simulink model "ssc_Probes_test_all_16a"  (R2019b)
settings: Solver=ode23t  StartTime=0.0  StopTime=10.0  RelTol=1e-3  EnableMultiTasking=on
undefined symbols (not defined in the file): damping_coeff
libraries: fl_lib x88, nesl_utility x71, Pneumatic_lib x16, fl_ps_legacy_lib x1
(part 3 of 4)

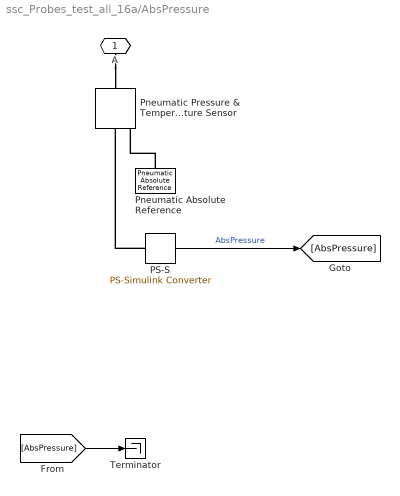
== system ssc_Probes_test_all_16a/AbsPressure ==
  PS-S : nesl_utility/PS-Simulink Converter  PhysicalDomain=network_engine_domain  SubClassName=ps_output  LeftPortType=input  RightPortType=output  PseudoPeriodic=off  Frequencies=[]  Unit=Pa  AffineConversion=off
  Pneumatic Absolute Reference : Pneumatic_lib/Pneumatic Elements/Pneumatic Absolute Reference
      settings: InternalSimscapePortConfiguration="{\"Bottom\":[],\"Left\":[{\"id\":\"A\",\"label\":\"\",\"type\":\"foundation.pneumatic.pneumatic\"}],\"Right\":[],\"Top\":[]}"
  Pneumatic Pressure & Temperature Sensor : Pneumatic_lib/Pneumatic Sensors/Pneumatic Pressure & Temperature Sensor
      settings: InternalSimscapePortConfiguration="{\"Bottom\":[],\"Left\":[{\"id\":\"A\",\"label\":\"A\",\"type\":\"foundation.pneumatic.pneumatic\"}],\"Right\":[{\"id\":\"B\",\"label\":\"B\",\"type\":\"foundation.pneumatic.pneumatic\"},{\"id\":\"P_ps\",\"label\":\"P\",\"type\":\"output\"},{\"id\":\"T_ps\",\"label\":\"T\",\"type\":\"output\"}],\"Top\":[]}"
  Terminator : Terminator
  A : PMIOPort  Side=Left
  wires:
  [AbsPressure] -> Terminator/1
  PS-S/1 -> [AbsPressure]  "AbsPressure"
  connections:
  PS-S/LConn1 -- Pneumatic Pressure & Temperature Sensor/RConn2
  Pneumatic Absolute Reference/LConn1 -- Pneumatic Pressure & Temperature Sensor/RConn1
  A/RConn1 -- Pneumatic Pressure & Temperature Sensor/LConn1

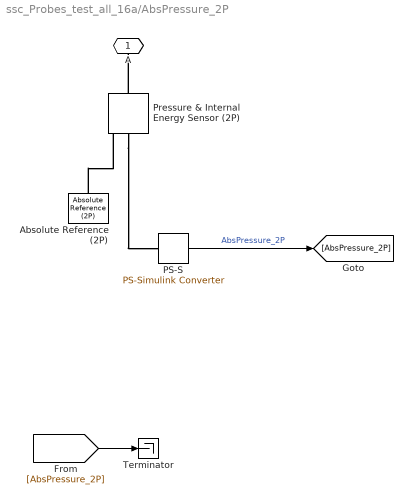
== system ssc_Probes_test_all_16a/AbsPressure_2P ==
  Absolute Reference (2P) : fl_lib/Two-Phase Fluid/Elements/Absolute Reference (2P)
      settings: SourceProductName=Simscape  SourceProductBaseCode=SS
  PS-S : nesl_utility/PS-Simulink Converter  PhysicalDomain=network_engine_domain  SubClassName=ps_output  LeftPortType=input  RightPortType=output  PseudoPeriodic=off  Frequencies=[]  Unit=Pa  AffineConversion=off
  Pressure & Internal Energy Sensor (2P) : fl_lib/Two-Phase Fluid/Sensors/Pressure & Internal Energy Sensor (2P)
      settings: SourceProductName=Simscape  SourceProductBaseCode=SS  InternalSimscapePortConfiguration="{\"Bottom\":[],\"Left\":[{\"id\":\"A\",\"label\":\"A\",\"type\":\"foundation.two_phase_fluid.two_phase_fluid\"}],\"Right\":[{\"id\":\"B\",\"label\":\"B\",\"type\":\"foundation.two_phase_fluid.two_phase_fluid\"},{\"id\":\"P\",\"label\":\"P\",\"type\":\"output\"},{\"id\":\"U\",\"label\":\"U\",\"type\":\"output\"}],\"Top\":[]}"
  Terminator : Terminator
  A : PMIOPort  Side=Left
  wires:
  [AbsPressure_2P] -> Terminator/1
  PS-S/1 -> [AbsPressure_2P]  "AbsPressure_2P"
  connections:
  Absolute Reference (2P)/LConn1 -- Pressure & Internal Energy Sensor (2P)/RConn1
  Pressure & Internal Energy Sensor (2P)/RConn2 -- PS-S/LConn1
  Pressure & Internal Energy Sensor (2P)/LConn1 -- A/RConn1

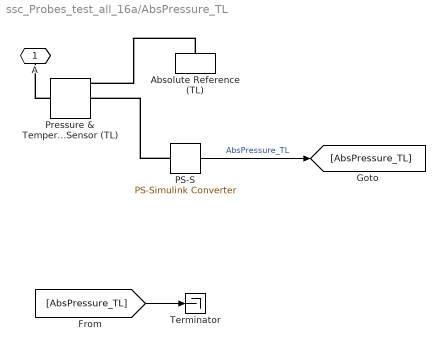
== system ssc_Probes_test_all_16a/AbsPressure_TL ==
  Absolute Reference (TL) : fl_lib/Thermal Liquid/Elements/Absolute Reference (TL)
      settings: SourceProductName=Simscape  SourceProductBaseCode=SS
  PS-S : nesl_utility/PS-Simulink Converter  PhysicalDomain=network_engine_domain  SubClassName=ps_output  LeftPortType=input  RightPortType=output  PseudoPeriodic=off  Frequencies=[]  Unit=Pa  AffineConversion=off
  Pressure & Temperature Sensor (TL) : fl_lib/Thermal Liquid/Sensors/Pressure & Temperature Sensor (TL)
      settings: SourceProductName=Simscape  SourceProductBaseCode=SS  InternalSimscapePortConfiguration="{\"Bottom\":[],\"Left\":[{\"id\":\"A\",\"label\":\"A\",\"type\":\"foundation.thermal_liquid.thermal_liquid\"}],\"Right\":[{\"id\":\"B\",\"label\":\"B\",\"type\":\"foundation.thermal_liquid.thermal_liquid\"},{\"id\":\"P\",\"label\":\"P\",\"type\":\"output\"},{\"id\":\"T\",\"label\":\"T\",\"type\":\"output\"}],\"Top\":[]}"
  Terminator : Terminator
  A : PMIOPort  Side=Left
  wires:
  [AbsPressure_TL] -> Terminator/1
  PS-S/1 -> [AbsPressure_TL]  "AbsPressure_TL"
  connections:
  PS-S/LConn1 -- Pressure & Temperature Sensor (TL)/RConn2
  Pressure & Temperature Sensor (TL)/LConn1 -- A/RConn1
  Absolute Reference (TL)/LConn1 -- Pressure & Temperature Sensor (TL)/RConn1

== system ssc_Probes_test_all_16a/AbsTemp_2P ==
  PS-S : nesl_utility/PS-Simulink Converter  PhysicalDomain=network_engine_domain  SubClassName=ps_output  LeftPortType=input  RightPortType=output  PseudoPeriodic=off  Frequencies=[]  Unit=K  AffineConversion=off
  Terminator : Terminator
  Thermodynamic Properties Sensor (2P) : fl_lib/Two-Phase Fluid/Sensors/Thermodynamic Properties Sensor (2P)
      settings: SourceProductName=Simscape  SourceProductBaseCode=SS  InternalSimscapePortConfiguration="{\"Bottom\":[],\"Left\":[{\"id\":\"A\",\"label\":\"A\",\"type\":\"foundation.two_phase_fluid.two_phase_fluid\"}],\"Right\":[{\"id\":\"T\",\"label\":\"T\",\"type\":\"output\"},{\"id\":\"H\",\"label\":\"h\",\"type\":\"output\"},{\"id\":\"V\",\"label\":\"v\",\"type\":\"output\"},{\"id\":\"S\",\"label\":\"s\",\"type\":\"output\"}],\"Top\":[]}"
  A : PMIOPort  Side=Left
  wires:
  PS-S/1 -> [AbsTemp_2P]  "AbsTemp_2P"
  [AbsTemp_2P] -> Terminator/1
  connections:
  A/RConn1 -- Thermodynamic Properties Sensor (2P)/LConn1
  Thermodynamic Properties Sensor (2P)/RConn1 -- PS-S/LConn1

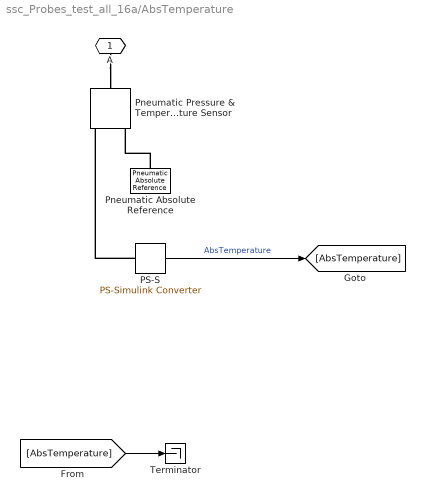
== system ssc_Probes_test_all_16a/AbsTemperature ==
  PS-S : nesl_utility/PS-Simulink Converter  PhysicalDomain=network_engine_domain  SubClassName=ps_output  LeftPortType=input  RightPortType=output  PseudoPeriodic=off  Frequencies=[]  Unit=K  AffineConversion=off
  Pneumatic Absolute Reference : Pneumatic_lib/Pneumatic Elements/Pneumatic Absolute Reference
      settings: InternalSimscapePortConfiguration="{\"Bottom\":[],\"Left\":[{\"id\":\"A\",\"label\":\"\",\"type\":\"foundation.pneumatic.pneumatic\"}],\"Right\":[],\"Top\":[]}"
  Pneumatic Pressure & Temperature Sensor : Pneumatic_lib/Pneumatic Sensors/Pneumatic Pressure & Temperature Sensor
      settings: InternalSimscapePortConfiguration="{\"Bottom\":[],\"Left\":[{\"id\":\"A\",\"label\":\"A\",\"type\":\"foundation.pneumatic.pneumatic\"}],\"Right\":[{\"id\":\"B\",\"label\":\"B\",\"type\":\"foundation.pneumatic.pneumatic\"},{\"id\":\"P_ps\",\"label\":\"P\",\"type\":\"output\"},{\"id\":\"T_ps\",\"label\":\"T\",\"type\":\"output\"}],\"Top\":[]}"
  Terminator : Terminator
  A : PMIOPort  Side=Left
  wires:
  [AbsTemperature] -> Terminator/1
  PS-S/1 -> [AbsTemperature]  "AbsTemperature"
  connections:
  A/RConn1 -- Pneumatic Pressure & Temperature Sensor/LConn1
  Pneumatic Absolute Reference/LConn1 -- Pneumatic Pressure & Temperature Sensor/RConn1
  PS-S/LConn1 -- Pneumatic Pressure & Temperature Sensor/RConn3

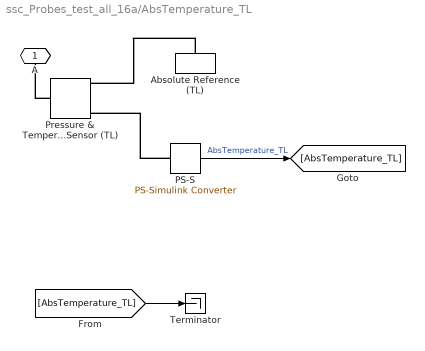
== system ssc_Probes_test_all_16a/AbsTemperature_TL ==
  Absolute Reference (TL) : fl_lib/Thermal Liquid/Elements/Absolute Reference (TL)
      settings: SourceProductName=Simscape  SourceProductBaseCode=SS
  PS-S : nesl_utility/PS-Simulink Converter  PhysicalDomain=network_engine_domain  SubClassName=ps_output  LeftPortType=input  RightPortType=output  PseudoPeriodic=off  Frequencies=[]  Unit=K  AffineConversion=off
  Pressure & Temperature Sensor (TL) : fl_lib/Thermal Liquid/Sensors/Pressure & Temperature Sensor (TL)
      settings: SourceProductName=Simscape  SourceProductBaseCode=SS  InternalSimscapePortConfiguration="{\"Bottom\":[],\"Left\":[{\"id\":\"A\",\"label\":\"A\",\"type\":\"foundation.thermal_liquid.thermal_liquid\"}],\"Right\":[{\"id\":\"B\",\"label\":\"B\",\"type\":\"foundation.thermal_liquid.thermal_liquid\"},{\"id\":\"P\",\"label\":\"P\",\"type\":\"output\"},{\"id\":\"T\",\"label\":\"T\",\"type\":\"output\"}],\"Top\":[]}"
  Terminator : Terminator
  A : PMIOPort  Side=Left
  wires:
  PS-S/1 -> [AbsTemperature_TL]  "AbsTemperature_TL"
  [AbsTemperature_TL] -> Terminator/1
  connections:
  Absolute Reference (TL)/LConn1 -- Pressure & Temperature Sensor (TL)/RConn1
  Pressure & Temperature Sensor (TL)/LConn1 -- A/RConn1
  PS-S/LConn1 -- Pressure & Temperature Sensor (TL)/RConn3

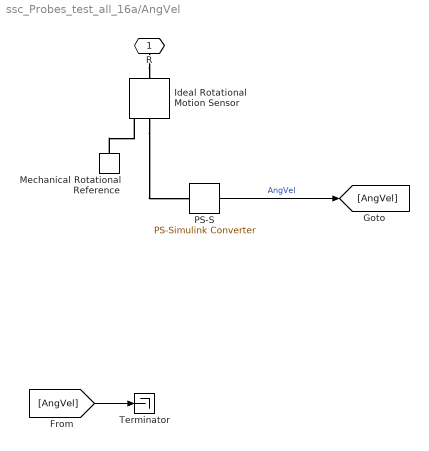
== system ssc_Probes_test_all_16a/AngVel ==
  Ideal Rotational Motion Sensor : fl_lib/Mechanical/Mechanical Sensors/Ideal Rotational Motion Sensor  offset=0 rad
  Mechanical Rotational Reference : fl_lib/Mechanical/Rotational Elements/Mechanical Rotational Reference
  PS-S : nesl_utility/PS-Simulink Converter  PhysicalDomain=network_engine_domain  SubClassName=ps_output  LeftPortType=input  RightPortType=output  PseudoPeriodic=off  Frequencies=[]  Unit=rad/s  AffineConversion=off
  Terminator : Terminator
  R : PMIOPort  Side=Left
  wires:
  [AngVel] -> Terminator/1
  PS-S/1 -> [AngVel]  "AngVel"
  connections:
  R/RConn1 -- Ideal Rotational Motion Sensor/LConn1
  Mechanical Rotational Reference/LConn1 -- Ideal Rotational Motion Sensor/RConn1
  Ideal Rotational Motion Sensor/RConn2 -- PS-S/LConn1

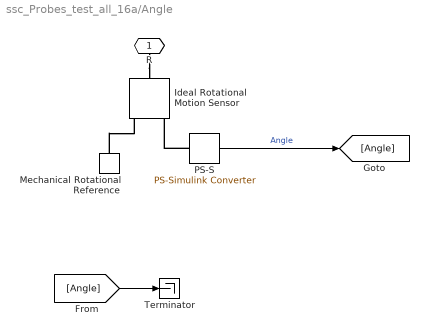
== system ssc_Probes_test_all_16a/Angle ==
  Ideal Rotational Motion Sensor : fl_lib/Mechanical/Mechanical Sensors/Ideal Rotational Motion Sensor  offset=0 rad
  Mechanical Rotational Reference : fl_lib/Mechanical/Rotational Elements/Mechanical Rotational Reference
  PS-S : nesl_utility/PS-Simulink Converter  PhysicalDomain=network_engine_domain  SubClassName=ps_output  LeftPortType=input  RightPortType=output  PseudoPeriodic=off  Frequencies=[]  Unit=rad  AffineConversion=off
  Terminator : Terminator
  R : PMIOPort  Side=Left
  wires:
  [Angle] -> Terminator/1
  PS-S/1 -> [Angle]  "Angle"
  connections:
  PS-S/LConn1 -- Ideal Rotational Motion Sensor/RConn3
  Mechanical Rotational Reference/LConn1 -- Ideal Rotational Motion Sensor/RConn1
  R/RConn1 -- Ideal Rotational Motion Sensor/LConn1

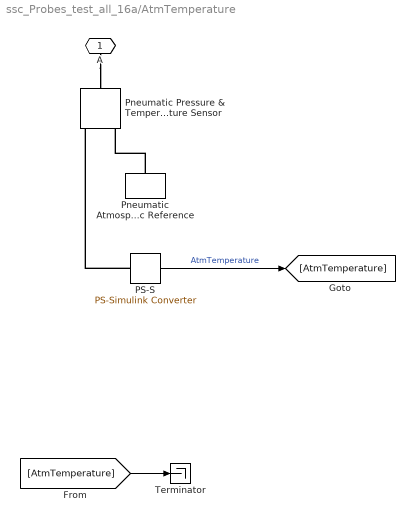
== system ssc_Probes_test_all_16a/AtmTemperature ==
  PS-S : nesl_utility/PS-Simulink Converter  PhysicalDomain=network_engine_domain  SubClassName=ps_output  LeftPortType=input  RightPortType=output  PseudoPeriodic=off  Frequencies=[]  Unit=K  AffineConversion=off
  Pneumatic Atmospheric Reference : Pneumatic_lib/Pneumatic Elements/Pneumatic Atmospheric Reference
      settings: InternalSimscapePortConfiguration="{\"Bottom\":[],\"Left\":[{\"id\":\"A\",\"label\":\"\",\"type\":\"foundation.pneumatic.pneumatic\"}],\"Right\":[],\"Top\":[]}"
  Pneumatic Pressure & Temperature Sensor : Pneumatic_lib/Pneumatic Sensors/Pneumatic Pressure & Temperature Sensor
      settings: InternalSimscapePortConfiguration="{\"Bottom\":[],\"Left\":[{\"id\":\"A\",\"label\":\"A\",\"type\":\"foundation.pneumatic.pneumatic\"}],\"Right\":[{\"id\":\"B\",\"label\":\"B\",\"type\":\"foundation.pneumatic.pneumatic\"},{\"id\":\"P_ps\",\"label\":\"P\",\"type\":\"output\"},{\"id\":\"T_ps\",\"label\":\"T\",\"type\":\"output\"}],\"Top\":[]}"
  Terminator : Terminator
  A : PMIOPort  Side=Left
  wires:
  [AtmTemperature] -> Terminator/1
  PS-S/1 -> [AtmTemperature]  "AtmTemperature"
  connections:
  PS-S/LConn1 -- Pneumatic Pressure & Temperature Sensor/RConn3
  Pneumatic Atmospheric Reference/LConn1 -- Pneumatic Pressure & Temperature Sensor/RConn1
  A/RConn1 -- Pneumatic Pressure & Temperature Sensor/LConn1

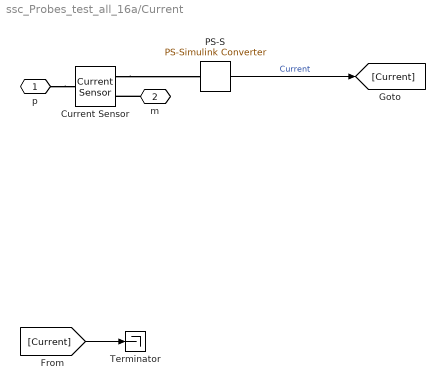
== system ssc_Probes_test_all_16a/Current ==
  Current Sensor : fl_lib/Electrical/Electrical Sensors/Current Sensor
  PS-S : nesl_utility/PS-Simulink Converter  PhysicalDomain=network_engine_domain  SubClassName=ps_output  LeftPortType=input  RightPortType=output  PseudoPeriodic=off  Frequencies=[]  Unit=A  AffineConversion=off
  Terminator : Terminator
  p : PMIOPort  Side=Left
  m : PMIOPort  Port=2  Side=Right
  wires:
  [Current] -> Terminator/1
  PS-S/1 -> [Current]  "Current"
  connections:
  Current Sensor/RConn1 -- PS-S/LConn1
  p/RConn1 -- Current Sensor/LConn1
  m/RConn1 -- Current Sensor/RConn2

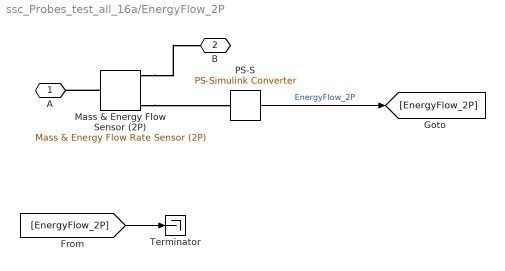
== system ssc_Probes_test_all_16a/EnergyFlow_2P ==
  Mass & Energy Flow Sensor (2P) : fl_lib/Two-Phase Fluid/Sensors/Mass & Energy Flow Rate Sensor (2P)
      settings: SourceProductName=Simscape  SourceProductBaseCode=SS  InternalSimscapePortConfiguration="{\"Bottom\":[],\"Left\":[{\"id\":\"A\",\"label\":\"A\",\"type\":\"foundation.two_phase_fluid.two_phase_fluid\"}],\"Right\":[{\"id\":\"B\",\"label\":\"B\",\"type\":\"foundation.two_phase_fluid.two_phase_fluid\"},{\"id\":\"M\",\"label\":\"M\",\"type\":\"output\"},{\"id\":\"PHI\",\"label\":\"Phi\",\"type\":\"output\"}],\"Top\":[]}"
  PS-S : nesl_utility/PS-Simulink Converter  PhysicalDomain=network_engine_domain  SubClassName=ps_output  LeftPortType=input  RightPortType=output  PseudoPeriodic=off  Frequencies=[]  Unit=kW  AffineConversion=off
  Terminator : Terminator
  A : PMIOPort  Side=Left
  B : PMIOPort  Port=2  Side=Right
  wires:
  [EnergyFlow_2P] -> Terminator/1
  PS-S/1 -> [EnergyFlow_2P]  "EnergyFlow_2P"
  connections:
  Mass & Energy Flow Sensor (2P)/RConn1 -- B/RConn1
  Mass & Energy Flow Sensor (2P)/RConn3 -- PS-S/LConn1
  Mass & Energy Flow Sensor (2P)/LConn1 -- A/RConn1

== system ssc_Probes_test_all_16a/Enthalpy_2P ==
  PS-S : nesl_utility/PS-Simulink Converter  PhysicalDomain=network_engine_domain  SubClassName=ps_output  LeftPortType=input  RightPortType=output  PseudoPeriodic=off  Frequencies=[]  Unit=kJ/kg  AffineConversion=off
  Terminator : Terminator
  Thermodynamic Properties Sensor (2P) : fl_lib/Two-Phase Fluid/Sensors/Thermodynamic Properties Sensor (2P)
      settings: SourceProductName=Simscape  SourceProductBaseCode=SS  InternalSimscapePortConfiguration="{\"Bottom\":[],\"Left\":[{\"id\":\"A\",\"label\":\"A\",\"type\":\"foundation.two_phase_fluid.two_phase_fluid\"}],\"Right\":[{\"id\":\"T\",\"label\":\"T\",\"type\":\"output\"},{\"id\":\"H\",\"label\":\"h\",\"type\":\"output\"},{\"id\":\"V\",\"label\":\"v\",\"type\":\"output\"},{\"id\":\"S\",\"label\":\"s\",\"type\":\"output\"}],\"Top\":[]}"
  A : PMIOPort  Side=Left
  wires:
  [Enthalpy_2P] -> Terminator/1
  PS-S/1 -> [Enthalpy_2P]  "Enthalpy_2P"
  connections:
  Thermodynamic Properties Sensor (2P)/RConn2 -- PS-S/LConn1
  A/RConn1 -- Thermodynamic Properties Sensor (2P)/LConn1

== system ssc_Probes_test_all_16a/Flow ==
  Ideal Hydraulic Flow Rate Sensor : fl_lib/Hydraulic/Hydraulic Sensors/Hydraulic Flow Rate Sensor
      settings: SourceProductName=Simscape
  PS-S : nesl_utility/PS-Simulink Converter  PhysicalDomain=network_engine_domain  SubClassName=ps_output  LeftPortType=input  RightPortType=output  PseudoPeriodic=off  Frequencies=[]  Unit=m^3/s  AffineConversion=off
  Terminator : Terminator
  A : PMIOPort  Side=Left
  B : PMIOPort  Port=2  Side=Right
  wires:
  [Flow] -> Terminator/1
  PS-S/1 -> [Flow]  "Flow"
  connections:
  A/RConn1 -- Ideal Hydraulic Flow Rate Sensor/LConn1
  Ideal Hydraulic Flow Rate Sensor/RConn1 -- PS-S/LConn1
  B/RConn1 -- Ideal Hydraulic Flow Rate Sensor/RConn2

== system ssc_Probes_test_all_16a/Flux ==
  Flux Sensor : fl_lib/Magnetic/Magnetic Sensors/Flux Sensor
      settings: SourceProductName=Simscape  SourceProductBaseCode=SS  InternalSimscapePortConfiguration="{\"Bottom\":[],\"Left\":[{\"id\":\"N\",\"label\":\"N\",\"type\":\"foundation.magnetic.magnetic\"}],\"Right\":[{\"id\":\"PHI\",\"label\":\"\",\"type\":\"output\"},{\"id\":\"S\",\"label\":\"S\",\"type\":\"foundation.magnetic.magnetic\"}],\"Top\":[]}"
  PS-S : nesl_utility/PS-Simulink Converter  PhysicalDomain=network_engine_domain  SubClassName=ps_output  LeftPortType=input  RightPortType=output  PseudoPeriodic=off  Frequencies=[]  Unit=Wb  AffineConversion=off
  Terminator : Terminator
  N : PMIOPort  Side=Left
  S : PMIOPort  Port=2  Side=Right
  wires:
  [Flux] -> Terminator/1
  PS-S/1 -> [Flux]  "Flux"
  connections:
  S/RConn1 -- Flux Sensor/RConn2
  Flux Sensor/RConn1 -- PS-S/LConn1
  N/RConn1 -- Flux Sensor/LConn1

== system ssc_Probes_test_all_16a/Force ==
  Ideal Force Sensor : fl_lib/Mechanical/Mechanical Sensors/Ideal Force Sensor
  PS-S : nesl_utility/PS-Simulink Converter  PhysicalDomain=network_engine_domain  SubClassName=ps_output  LeftPortType=input  RightPortType=output  PseudoPeriodic=off  Frequencies=[]  Unit=N  AffineConversion=off
  Terminator : Terminator
  R : PMIOPort  Side=Left
  C : PMIOPort  Port=2  Side=Right
  wires:
  [Force] -> Terminator/1
  PS-S/1 -> [Force]  "Force"
  connections:
  R/RConn1 -- Ideal Force Sensor/LConn1
  Ideal Force Sensor/RConn2 -- PS-S/LConn1
  C/RConn1 -- Ideal Force Sensor/RConn1

== system ssc_Probes_test_all_16a/GasHeatFlow ==
  PS-S : nesl_utility/PS-Simulink Converter  PhysicalDomain=network_engine_domain  SubClassName=ps_output  LeftPortType=input  RightPortType=output  PseudoPeriodic=off  Frequencies=[]  Unit=J/s  AffineConversion=off
  Pneumatic Mass & Heat Flow Sensor : Pneumatic_lib/Pneumatic Sensors/Pneumatic Mass & Heat Flow Sensor
      settings: InternalSimscapePortConfiguration="{\"Bottom\":[],\"Left\":[{\"id\":\"A\",\"label\":\"A\",\"type\":\"foundation.pneumatic.pneumatic\"}],\"Right\":[{\"id\":\"B\",\"label\":\"B\",\"type\":\"foundation.pneumatic.pneumatic\"},{\"id\":\"G_ps\",\"label\":\"G\",\"type\":\"output\"},{\"id\":\"Q_ps\",\"label\":\"Q\",\"type\":\"output\"}],\"Top\":[]}"
  Terminator : Terminator
  A : PMIOPort  Side=Left
  B : PMIOPort  Port=2  Side=Right
  wires:
  [GasHeatFlow] -> Terminator/1
  PS-S/1 -> [GasHeatFlow]  "GasHeatFlow"
  connections:
  A/RConn1 -- Pneumatic Mass & Heat Flow Sensor/LConn1
  B/RConn1 -- Pneumatic Mass & Heat Flow Sensor/RConn1
  PS-S/LConn1 -- Pneumatic Mass & Heat Flow Sensor/RConn3

== system ssc_Probes_test_all_16a/GaugePressure ==
  PS-S : nesl_utility/PS-Simulink Converter  PhysicalDomain=network_engine_domain  SubClassName=ps_output  LeftPortType=input  RightPortType=output  PseudoPeriodic=off  Frequencies=[]  Unit=Pa  AffineConversion=off
  Pneumatic Atmospheric Reference : Pneumatic_lib/Pneumatic Elements/Pneumatic Atmospheric Reference
      settings: InternalSimscapePortConfiguration="{\"Bottom\":[],\"Left\":[{\"id\":\"A\",\"label\":\"\",\"type\":\"foundation.pneumatic.pneumatic\"}],\"Right\":[],\"Top\":[]}"
  Pneumatic Pressure & Temperature Sensor : Pneumatic_lib/Pneumatic Sensors/Pneumatic Pressure & Temperature Sensor
      settings: InternalSimscapePortConfiguration="{\"Bottom\":[],\"Left\":[{\"id\":\"A\",\"label\":\"A\",\"type\":\"foundation.pneumatic.pneumatic\"}],\"Right\":[{\"id\":\"B\",\"label\":\"B\",\"type\":\"foundation.pneumatic.pneumatic\"},{\"id\":\"P_ps\",\"label\":\"P\",\"type\":\"output\"},{\"id\":\"T_ps\",\"label\":\"T\",\"type\":\"output\"}],\"Top\":[]}"
  Terminator : Terminator
  A : PMIOPort  Side=Left
  wires:
  [GaugePressure] -> Terminator/1
  PS-S/1 -> [GaugePressure]  "GaugePressure"
  connections:
  A/RConn1 -- Pneumatic Pressure & Temperature Sensor/LConn1
  Pneumatic Atmospheric Reference/LConn1 -- Pneumatic Pressure & Temperature Sensor/RConn1
  PS-S/LConn1 -- Pneumatic Pressure & Temperature Sensor/RConn2

== system ssc_Probes_test_all_16a/HeatFlow ==
  Ideal Heat Flow Sensor : fl_lib/Thermal/Thermal Sensors/Heat Flow Rate Sensor
      settings: SourceProductName=Simscape  SourceProductBaseCode=SS
  PS-S : nesl_utility/PS-Simulink Converter  PhysicalDomain=network_engine_domain  SubClassName=ps_output  LeftPortType=input  RightPortType=output  PseudoPeriodic=off  Frequencies=[]  Unit=J/s  AffineConversion=off
  Terminator : Terminator
  A : PMIOPort  Side=Left
  B : PMIOPort  Port=2  Side=Right
  wires:
  [HeatFlow] -> Terminator/1
  PS-S/1 -> [HeatFlow]  "HeatFlow"
  connections:
  B/RConn1 -- Ideal Heat Flow Sensor/RConn2
  Ideal Heat Flow Sensor/RConn1 -- PS-S/LConn1
  A/RConn1 -- Ideal Heat Flow Sensor/LConn1

== system ssc_Probes_test_all_16a/InternalEnergy_2P ==
  Absolute Reference (2P) : fl_lib/Two-Phase Fluid/Elements/Absolute Reference (2P)
      settings: SourceProductName=Simscape  SourceProductBaseCode=SS
  PS-S : nesl_utility/PS-Simulink Converter  PhysicalDomain=network_engine_domain  SubClassName=ps_output  LeftPortType=input  RightPortType=output  PseudoPeriodic=off  Frequencies=[]  Unit=kJ/kg  AffineConversion=off
  Pressure & Internal Energy Sensor (2P) : fl_lib/Two-Phase Fluid/Sensors/Pressure & Internal Energy Sensor (2P)
      settings: SourceProductName=Simscape  SourceProductBaseCode=SS  InternalSimscapePortConfiguration="{\"Bottom\":[],\"Left\":[{\"id\":\"A\",\"label\":\"A\",\"type\":\"foundation.two_phase_fluid.two_phase_fluid\"}],\"Right\":[{\"id\":\"B\",\"label\":\"B\",\"type\":\"foundation.two_phase_fluid.two_phase_fluid\"},{\"id\":\"P\",\"label\":\"P\",\"type\":\"output\"},{\"id\":\"U\",\"label\":\"U\",\"type\":\"output\"}],\"Top\":[]}"
  Terminator : Terminator
  A : PMIOPort  Side=Left
  wires:
  PS-S/1 -> [InternalEnergy_2P]  "InternalEnergy_2P"
  [InternalEnergy_2P] -> Terminator/1
  connections:
  Pressure & Internal Energy Sensor (2P)/LConn1 -- A/RConn1
  Pressure & Internal Energy Sensor (2P)/RConn3 -- PS-S/LConn1
  Absolute Reference (2P)/LConn1 -- Pressure & Internal Energy Sensor (2P)/RConn1

== system ssc_Probes_test_all_16a/MMF ==
  MMF Sensor : fl_lib/Magnetic/Magnetic Sensors/MMF Sensor
      settings: SourceProductName=Simscape  SourceProductBaseCode=SS  InternalSimscapePortConfiguration="{\"Bottom\":[],\"Left\":[{\"id\":\"N\",\"label\":\"N\",\"type\":\"foundation.magnetic.magnetic\"}],\"Right\":[{\"id\":\"MMF\",\"label\":\"\",\"type\":\"output\"},{\"id\":\"S\",\"label\":\"S\",\"type\":\"foundation.magnetic.magnetic\"}],\"Top\":[]}"
  Magnetic Reference : fl_lib/Magnetic/Magnetic Elements/Magnetic Reference
      settings: SourceProductName=Simscape  SourceProductBaseCode=SS  InternalSimscapePortConfiguration="{\"Bottom\":[],\"Left\":[{\"id\":\"M\",\"label\":\"\",\"type\":\"foundation.magnetic.magnetic\"}],\"Right\":[],\"Top\":[]}"
  PS-S : nesl_utility/PS-Simulink Converter  PhysicalDomain=network_engine_domain  SubClassName=ps_output  LeftPortType=input  RightPortType=output  PseudoPeriodic=off  Frequencies=[]  Unit=A  AffineConversion=off
  Terminator : Terminator
  N : PMIOPort  Side=Left
  wires:
  [MMF] -> Terminator/1
  PS-S/1 -> [MMF]  "MMF"
  connections:
  N/RConn1 -- MMF Sensor/LConn1
  MMF Sensor/RConn1 -- PS-S/LConn1
  Magnetic Reference/LConn1 -- MMF Sensor/RConn2

== system ssc_Probes_test_all_16a/MassFlow ==
  PS-S : nesl_utility/PS-Simulink Converter  PhysicalDomain=network_engine_domain  SubClassName=ps_output  LeftPortType=input  RightPortType=output  PseudoPeriodic=off  Frequencies=[]  Unit=kg/s  AffineConversion=off
  Pneumatic Mass & Heat Flow Sensor : Pneumatic_lib/Pneumatic Sensors/Pneumatic Mass & Heat Flow Sensor
      settings: InternalSimscapePortConfiguration="{\"Bottom\":[],\"Left\":[{\"id\":\"A\",\"label\":\"A\",\"type\":\"foundation.pneumatic.pneumatic\"}],\"Right\":[{\"id\":\"B\",\"label\":\"B\",\"type\":\"foundation.pneumatic.pneumatic\"},{\"id\":\"G_ps\",\"label\":\"G\",\"type\":\"output\"},{\"id\":\"Q_ps\",\"label\":\"Q\",\"type\":\"output\"}],\"Top\":[]}"
  Terminator : Terminator
  A : PMIOPort  Side=Left
  B : PMIOPort  Port=2  Side=Right
  wires:
  [MassFlow] -> Terminator/1
  PS-S/1 -> [MassFlow]  "MassFlow"
  connections:
  B/RConn1 -- Pneumatic Mass & Heat Flow Sensor/RConn1
  Pneumatic Mass & Heat Flow Sensor/RConn2 -- PS-S/LConn1
  A/RConn1 -- Pneumatic Mass & Heat Flow Sensor/LConn1

== system ssc_Probes_test_all_16a/MassFlow_2P ==
  Mass & Energy Flow Sensor (2P) : fl_lib/Two-Phase Fluid/Sensors/Mass & Energy Flow Rate Sensor (2P)
      settings: SourceProductName=Simscape  SourceProductBaseCode=SS  InternalSimscapePortConfiguration="{\"Bottom\":[],\"Left\":[{\"id\":\"A\",\"label\":\"A\",\"type\":\"foundation.two_phase_fluid.two_phase_fluid\"}],\"Right\":[{\"id\":\"B\",\"label\":\"B\",\"type\":\"foundation.two_phase_fluid.two_phase_fluid\"},{\"id\":\"M\",\"label\":\"M\",\"type\":\"output\"},{\"id\":\"PHI\",\"label\":\"Phi\",\"type\":\"output\"}],\"Top\":[]}"
  PS-S : nesl_utility/PS-Simulink Converter  PhysicalDomain=network_engine_domain  SubClassName=ps_output  LeftPortType=input  RightPortType=output  PseudoPeriodic=off  Frequencies=[]  Unit=kg/s  AffineConversion=off
  Terminator : Terminator
  A : PMIOPort  Side=Left
  B : PMIOPort  Port=2  Side=Right
  wires:
  PS-S/1 -> [MassFlow_2P]  "MassFlow_2P"
  [MassFlow_2P] -> Terminator/1
  connections:
  Mass & Energy Flow Sensor (2P)/LConn1 -- A/RConn1
  Mass & Energy Flow Sensor (2P)/RConn2 -- PS-S/LConn1
  Mass & Energy Flow Sensor (2P)/RConn1 -- B/RConn1

== system ssc_Probes_test_all_16a/MassFlow_TL ==
  Mass Flow Rate & Thermal Flux Sensor (TL) : fl_lib/Thermal Liquid/Sensors/Mass & Energy Flow Rate Sensor (TL)
      settings: SourceProductName=Simscape  SourceProductBaseCode=SS  InternalSimscapePortConfiguration="{\"Bottom\":[],\"Left\":[{\"id\":\"A\",\"label\":\"A\",\"type\":\"foundation.thermal_liquid.thermal_liquid\"}],\"Right\":[{\"id\":\"B\",\"label\":\"B\",\"type\":\"foundation.thermal_liquid.thermal_liquid\"},{\"id\":\"M\",\"label\":\"M\",\"type\":\"output\"},{\"id\":\"PHI\",\"label\":\"Phi\",\"type\":\"output\"}],\"Top\":[]}"
  PS-S : nesl_utility/PS-Simulink Converter  PhysicalDomain=network_engine_domain  SubClassName=ps_output  LeftPortType=input  RightPortType=output  PseudoPeriodic=off  Frequencies=[]  Unit=kg/s  AffineConversion=off
  Terminator : Terminator
  A : PMIOPort  Side=Left
  B : PMIOPort  Port=2  Side=Right
  wires:
  PS-S/1 -> [MassFlow_TL]  "MassFlow_TL"
  [MassFlow_TL] -> Terminator/1
  connections:
  Mass Flow Rate & Thermal Flux Sensor (TL)/LConn1 -- A/RConn1
  PS-S/LConn1 -- Mass Flow Rate & Thermal Flux Sensor (TL)/RConn2
  Mass Flow Rate & Thermal Flux Sensor (TL)/RConn1 -- B/RConn1

== system ssc_Probes_test_all_16a/PhysicalSignal ==
  PS Gain : fl_ps_legacy_lib/Legacy Physical Signals/Functions/PS Gain  gain=1
      settings: SourceProductName=Simscape
  PS-S : nesl_utility/PS-Simulink Converter  PhysicalDomain=network_engine_domain  SubClassName=ps_output  LeftPortType=input  RightPortType=output  PseudoPeriodic=off  Frequencies=[]  Unit=1  AffineConversion=off
  Terminator : Terminator
  PS : PMIOPort  Side=Left
  wires:
  [PhysicalSignal] -> Terminator/1
  PS-S/1 -> [PhysicalSignal]  "PhysicalSignal"
  connections:
  PS Gain/LConn1 -- PS/RConn1
  PS Gain/RConn1 -- PS-S/LConn1

== system ssc_Probes_test_all_16a/Position ==
  Ideal Translational Motion Sensor : fl_lib/Mechanical/Mechanical Sensors/Ideal Translational Motion Sensor  offset=0 m
  Mechanical Translational Reference : fl_lib/Mechanical/Translational Elements/Mechanical Translational Reference
  PS-S : nesl_utility/PS-Simulink Converter  PhysicalDomain=network_engine_domain  SubClassName=ps_output  LeftPortType=input  RightPortType=output  PseudoPeriodic=off  Frequencies=[]  Unit=m  AffineConversion=off
  Terminator : Terminator
  R : PMIOPort  Side=Left
  wires:
  [Position] -> Terminator/1
  PS-S/1 -> [Position]  "Position"
  connections:
  R/RConn1 -- Ideal Translational Motion Sensor/LConn1
  Mechanical Translational Reference/LConn1 -- Ideal Translational Motion Sensor/RConn1
  PS-S/LConn1 -- Ideal Translational Motion Sensor/RConn3

== system ssc_Probes_test_all_16a/Pressure ==
  Hydraulic Reference : fl_lib/Hydraulic/Hydraulic Elements/Hydraulic Reference
      settings: SourceProductName=Simscape
  Ideal Hydraulic Pressure Sensor : fl_lib/Hydraulic/Hydraulic Sensors/Hydraulic Pressure Sensor
      settings: SourceProductName=Simscape
  PS-S : nesl_utility/PS-Simulink Converter  PhysicalDomain=network_engine_domain  SubClassName=ps_output  LeftPortType=input  RightPortType=output  PseudoPeriodic=off  Frequencies=[]  Unit=Pa  AffineConversion=off
  Terminator : Terminator
  A : PMIOPort  Side=Left
  wires:
  [Pressure] -> Terminator/1
  PS-S/1 -> [Pressure]  "Pressure"
  connections:
  A/RConn1 -- Ideal Hydraulic Pressure Sensor/LConn1
  Hydraulic Reference/LConn1 -- Ideal Hydraulic Pressure Sensor/RConn1
  PS-S/LConn1 -- Ideal Hydraulic Pressure Sensor/RConn2

== system ssc_Probes_test_all_16a/SpecificVol_2P ==
  PS-S : nesl_utility/PS-Simulink Converter  PhysicalDomain=network_engine_domain  SubClassName=ps_output  LeftPortType=input  RightPortType=output  PseudoPeriodic=off  Frequencies=[]  Unit=m^3/kg  AffineConversion=off
  Terminator : Terminator
  Thermodynamic Properties Sensor (2P) : fl_lib/Two-Phase Fluid/Sensors/Thermodynamic Properties Sensor (2P)
      settings: SourceProductName=Simscape  SourceProductBaseCode=SS  InternalSimscapePortConfiguration="{\"Bottom\":[],\"Left\":[{\"id\":\"A\",\"label\":\"A\",\"type\":\"foundation.two_phase_fluid.two_phase_fluid\"}],\"Right\":[{\"id\":\"T\",\"label\":\"T\",\"type\":\"output\"},{\"id\":\"H\",\"label\":\"h\",\"type\":\"output\"},{\"id\":\"V\",\"label\":\"v\",\"type\":\"output\"},{\"id\":\"S\",\"label\":\"s\",\"type\":\"output\"}],\"Top\":[]}"
  A : PMIOPort  Side=Left
  wires:
  PS-S/1 -> [SpecificVol_2P]  "SpecificVol_2P"
  [SpecificVol_2P] -> Terminator/1
  connections:
  A/RConn1 -- Thermodynamic Properties Sensor (2P)/LConn1
  Thermodynamic Properties Sensor (2P)/RConn3 -- PS-S/LConn1

== system ssc_Probes_test_all_16a/Temperature ==
  Ideal Temperature Sensor : fl_lib/Thermal/Thermal Sensors/Temperature Sensor
  PS-S : nesl_utility/PS-Simulink Converter  PhysicalDomain=network_engine_domain  SubClassName=ps_output  LeftPortType=input  RightPortType=output  PseudoPeriodic=off  Frequencies=[]  Unit=K  AffineConversion=off
  Terminator : Terminator
  Thermal Reference : fl_lib/Thermal/Thermal Elements/Thermal Reference
  A : PMIOPort  Side=Left
  wires:
  [Temperature] -> Terminator/1
  PS-S/1 -> [Temperature]  "Temperature"
  connections:
  PS-S/LConn1 -- Ideal Temperature Sensor/RConn2
  Thermal Reference/LConn1 -- Ideal Temperature Sensor/RConn1
  A/RConn1 -- Ideal Temperature Sensor/LConn1

== system ssc_Probes_test_all_16a/ThermalFlux_TL ==
  Mass Flow Rate & Thermal Flux Sensor (TL) : fl_lib/Thermal Liquid/Sensors/Mass & Energy Flow Rate Sensor (TL)
      settings: SourceProductName=Simscape  SourceProductBaseCode=SS  InternalSimscapePortConfiguration="{\"Bottom\":[],\"Left\":[{\"id\":\"A\",\"label\":\"A\",\"type\":\"foundation.thermal_liquid.thermal_liquid\"}],\"Right\":[{\"id\":\"B\",\"label\":\"B\",\"type\":\"foundation.thermal_liquid.thermal_liquid\"},{\"id\":\"M\",\"label\":\"M\",\"type\":\"output\"},{\"id\":\"PHI\",\"label\":\"Phi\",\"type\":\"output\"}],\"Top\":[]}"
  PS-S : nesl_utility/PS-Simulink Converter  PhysicalDomain=network_engine_domain  SubClassName=ps_output  LeftPortType=input  RightPortType=output  PseudoPeriodic=off  Frequencies=[]  Unit=J/s  AffineConversion=off
  Terminator : Terminator
  A : PMIOPort  Side=Left
  B : PMIOPort  Port=2  Side=Right
  wires:
  [ThermalFlux_TL] -> Terminator/1
  PS-S/1 -> [ThermalFlux_TL]  "ThermalFlux_TL"
  connections:
  Mass Flow Rate & Thermal Flux Sensor (TL)/RConn3 -- PS-S/LConn1
  Mass Flow Rate & Thermal Flux Sensor (TL)/RConn1 -- B/RConn1
  Mass Flow Rate & Thermal Flux Sensor (TL)/LConn1 -- A/RConn1

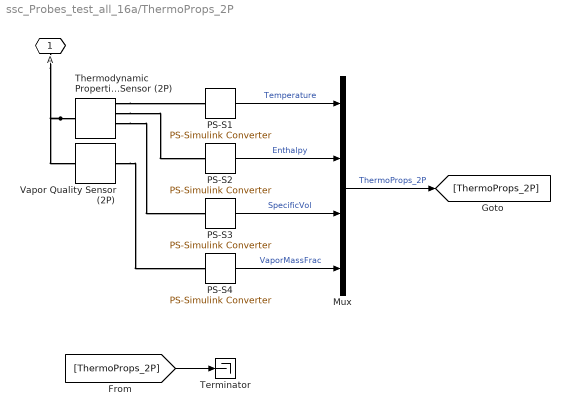
== system ssc_Probes_test_all_16a/ThermoProps_2P ==
  Mux : Mux
  PS-S1 : nesl_utility/PS-Simulink Converter  PhysicalDomain=network_engine_domain  SubClassName=ps_output  LeftPortType=input  RightPortType=output  PseudoPeriodic=off  Frequencies=[]  Unit=K  AffineConversion=off
  PS-S2 : nesl_utility/PS-Simulink Converter  PhysicalDomain=network_engine_domain  SubClassName=ps_output  LeftPortType=input  RightPortType=output  PseudoPeriodic=off  Frequencies=[]  Unit=kJ/kg  AffineConversion=off
  PS-S3 : nesl_utility/PS-Simulink Converter  PhysicalDomain=network_engine_domain  SubClassName=ps_output  LeftPortType=input  RightPortType=output  PseudoPeriodic=off  Frequencies=[]  Unit=m^3/kg  AffineConversion=off
  PS-S4 : nesl_utility/PS-Simulink Converter  PhysicalDomain=network_engine_domain  SubClassName=ps_output  LeftPortType=input  RightPortType=output  PseudoPeriodic=off  Frequencies=[]  Unit=1  AffineConversion=off
  Terminator : Terminator
  Thermodynamic Properties Sensor (2P) : fl_lib/Two-Phase Fluid/Sensors/Thermodynamic Properties Sensor (2P)
      settings: SourceProductName=Simscape  SourceProductBaseCode=SS  InternalSimscapePortConfiguration="{\"Bottom\":[],\"Left\":[{\"id\":\"A\",\"label\":\"A\",\"type\":\"foundation.two_phase_fluid.two_phase_fluid\"}],\"Right\":[{\"id\":\"T\",\"label\":\"T\",\"type\":\"output\"},{\"id\":\"H\",\"label\":\"h\",\"type\":\"output\"},{\"id\":\"V\",\"label\":\"v\",\"type\":\"output\"},{\"id\":\"S\",\"label\":\"s\",\"type\":\"output\"}],\"Top\":[]}"
  Vapor Quality Sensor (2P) : fl_lib/Two-Phase Fluid/Sensors/Vapor Quality Sensor (2P)  vapor_fraction_spec=foundation.enum.vapor_fraction_spec.quality
      settings: SourceProductName=Simscape  SourceProductBaseCode=SS  InternalSimscapePortConfiguration="{\"Bottom\":[],\"Left\":[{\"id\":\"A\",\"label\":\"A\",\"type\":\"foundation.two_phase_fluid.two_phase_fluid\"}],\"Right\":[{\"id\":\"X\",\"label\":\"X\",\"type\":\"output\"}],\"Top\":[]}"
  A : PMIOPort  Side=Left
  wires:
  Mux/1 -> [ThermoProps_2P]  "ThermoProps_2P"
  [ThermoProps_2P] -> Terminator/1
  PS-S1/1 -> Mux/1  "Temperature"
  PS-S2/1 -> Mux/2  "Enthalpy"
  PS-S3/1 -> Mux/3  "SpecificVol"
  PS-S4/1 -> Mux/4  "VaporMassFrac"
  connections:
  Thermodynamic Properties Sensor (2P)/LConn1 -- A/RConn1 -- Vapor Quality Sensor (2P)/LConn1
  Thermodynamic Properties Sensor (2P)/RConn1 -- PS-S1/LConn1
  Thermodynamic Properties Sensor (2P)/RConn2 -- PS-S2/LConn1
  Thermodynamic Properties Sensor (2P)/RConn3 -- PS-S3/LConn1
  Vapor Quality Sensor (2P)/RConn1 -- PS-S4/LConn1

== system ssc_Probes_test_all_16a/Torque ==
  Ideal Torque Sensor : fl_lib/Mechanical/Mechanical Sensors/Ideal Torque Sensor
  PS-S : nesl_utility/PS-Simulink Converter  PhysicalDomain=network_engine_domain  SubClassName=ps_output  LeftPortType=input  RightPortType=output  PseudoPeriodic=off  Frequencies=[]  Unit=N*m  AffineConversion=off
  Terminator : Terminator
  R : PMIOPort  Side=Left
  C : PMIOPort  Port=2  Side=Right
  wires:
  [Torque] -> Terminator/1
  PS-S/1 -> [Torque]  "Torque"
  connections:
  C/RConn1 -- Ideal Torque Sensor/RConn1
  Ideal Torque Sensor/RConn2 -- PS-S/LConn1
  R/RConn1 -- Ideal Torque Sensor/LConn1

== system ssc_Probes_test_all_16a/VaporMassFraction_2P ==
  PS-S : nesl_utility/PS-Simulink Converter  PhysicalDomain=network_engine_domain  SubClassName=ps_output  LeftPortType=input  RightPortType=output  PseudoPeriodic=off  Frequencies=[]  Unit=1  AffineConversion=off
  Terminator : Terminator
  Thermodynamic Properties Sensor (2P) : fl_lib/Two-Phase Fluid/Sensors/Thermodynamic Properties Sensor (2P)
      settings: SourceProductName=Simscape  SourceProductBaseCode=SS  InternalSimscapePortConfiguration="{\"Bottom\":[],\"Left\":[{\"id\":\"A\",\"label\":\"A\",\"type\":\"foundation.two_phase_fluid.two_phase_fluid\"}],\"Right\":[{\"id\":\"T\",\"label\":\"T\",\"type\":\"output\"},{\"id\":\"H\",\"label\":\"h\",\"type\":\"output\"},{\"id\":\"V\",\"label\":\"v\",\"type\":\"output\"},{\"id\":\"S\",\"label\":\"s\",\"type\":\"output\"}],\"Top\":[]}"
  Vapor Quality Sensor (2P) : fl_lib/Two-Phase Fluid/Sensors/Vapor Quality Sensor (2P)  vapor_fraction_spec=foundation.enum.vapor_fraction_spec.quality
      settings: SourceProductName=Simscape  SourceProductBaseCode=SS  InternalSimscapePortConfiguration="{\"Bottom\":[],\"Left\":[{\"id\":\"A\",\"label\":\"A\",\"type\":\"foundation.two_phase_fluid.two_phase_fluid\"}],\"Right\":[{\"id\":\"X\",\"label\":\"X\",\"type\":\"output\"}],\"Top\":[]}"
  A : PMIOPort  Side=Left
  wires:
  [VaporMassFraction_2P] -> Terminator/1
  PS-S/1 -> [VaporMassFraction_2P]  "VaporMassFraction_2P"
  connections:
  Thermodynamic Properties Sensor (2P)/LConn1 -- A/RConn1 -- Vapor Quality Sensor (2P)/LConn1
  Vapor Quality Sensor (2P)/RConn1 -- PS-S/LConn1

== system ssc_Probes_test_all_16a/Velocity ==
  Ideal Translational Motion Sensor : fl_lib/Mechanical/Mechanical Sensors/Ideal Translational Motion Sensor  offset=0 m
  Mechanical Translational Reference : fl_lib/Mechanical/Translational Elements/Mechanical Translational Reference
  PS-S : nesl_utility/PS-Simulink Converter  PhysicalDomain=network_engine_domain  SubClassName=ps_output  LeftPortType=input  RightPortType=output  PseudoPeriodic=off  Frequencies=[]  Unit=m/s  AffineConversion=off
  Terminator : Terminator
  R : PMIOPort  Side=Left
  wires:
  [Velocity] -> Terminator/1
  PS-S/1 -> [Velocity]  "Velocity"
  connections:
  Mechanical Translational Reference/LConn1 -- Ideal Translational Motion Sensor/RConn1
  R/RConn1 -- Ideal Translational Motion Sensor/LConn1
  Ideal Translational Motion Sensor/RConn2 -- PS-S/LConn1

== system ssc_Probes_test_all_16a/Voltage ==
  Electrical Reference : fl_lib/Electrical/Electrical Elements/Electrical Reference
  PS-S : nesl_utility/PS-Simulink Converter  PhysicalDomain=network_engine_domain  SubClassName=ps_output  LeftPortType=input  RightPortType=output  PseudoPeriodic=off  Frequencies=[]  Unit=V  AffineConversion=off
  Terminator : Terminator
  Voltage Sensor : fl_lib/Electrical/Electrical Sensors/Voltage Sensor
  p : PMIOPort  Side=Left
  wires:
  [Voltage] -> Terminator/1
  PS-S/1 -> [Voltage]  "Voltage"
  connections:
  p/RConn1 -- Voltage Sensor/LConn1
  PS-S/LConn1 -- Voltage Sensor/RConn1
  Electrical Reference/LConn1 -- Voltage Sensor/RConn2

== system ssc_Probes_test_all_16a/VolumetricFlow_2P ==
  PS-S : nesl_utility/PS-Simulink Converter  PhysicalDomain=network_engine_domain  SubClassName=ps_output  LeftPortType=input  RightPortType=output  PseudoPeriodic=off  Frequencies=[]  Unit=m^3/s  AffineConversion=off
  Terminator : Terminator
  Volumetric Flow Sensor (2P) : fl_lib/Two-Phase Fluid/Sensors/Volumetric Flow Rate Sensor (2P)
      settings: SourceProductName=Simscape  SourceProductBaseCode=SS  InternalSimscapePortConfiguration="{\"Bottom\":[],\"Left\":[{\"id\":\"A\",\"label\":\"A\",\"type\":\"foundation.two_phase_fluid.two_phase_fluid\"}],\"Right\":[{\"id\":\"B\",\"label\":\"B\",\"type\":\"foundation.two_phase_fluid.two_phase_fluid\"},{\"id\":\"V\",\"label\":\"V\",\"type\":\"output\"}],\"Top\":[]}"
  A : PMIOPort  Side=Left
  B : PMIOPort  Port=2  Side=Right
  wires:
  PS-S/1 -> [VolumetricFlow_2P]  "VolumetricFlow_2P"
  [VolumetricFlow_2P] -> Terminator/1
  connections:
  Volumetric Flow Sensor (2P)/LConn1 -- A/RConn1
  Volumetric Flow Sensor (2P)/RConn2 -- PS-S/LConn1
  Volumetric Flow Sensor (2P)/RConn1 -- B/RConn1

== system ssc_Probes_test_all_16a/dAngVel ==
  Ideal Rotational Motion Sensor : fl_lib/Mechanical/Mechanical Sensors/Ideal Rotational Motion Sensor  offset=0 rad
  PS-S : nesl_utility/PS-Simulink Converter  PhysicalDomain=network_engine_domain  SubClassName=ps_output  LeftPortType=input  RightPortType=output  PseudoPeriodic=off  Frequencies=[]  Unit=rad/s  AffineConversion=off
  Terminator : Terminator
  R : PMIOPort  Side=Left
  C : PMIOPort  Port=2  Side=Right
  wires:
  [dAngVel] -> Terminator/1
  PS-S/1 -> [dAngVel]  "dAngVel"
  connections:
  Ideal Rotational Motion Sensor/RConn2 -- PS-S/LConn1
  C/RConn1 -- Ideal Rotational Motion Sensor/RConn1
  R/RConn1 -- Ideal Rotational Motion Sensor/LConn1

== system ssc_Probes_test_all_16a/dAngle ==
  Ideal Rotational Motion Sensor : fl_lib/Mechanical/Mechanical Sensors/Ideal Rotational Motion Sensor  offset=0 rad
  PS-S : nesl_utility/PS-Simulink Converter  PhysicalDomain=network_engine_domain  SubClassName=ps_output  LeftPortType=input  RightPortType=output  PseudoPeriodic=off  Frequencies=[]  Unit=rad  AffineConversion=off
  Terminator : Terminator
  R : PMIOPort  Side=Left
  C : PMIOPort  Port=2  Side=Right
  wires:
  [dAngle] -> Terminator/1
  PS-S/1 -> [dAngle]  "dAngle"
  connections:
  R/RConn1 -- Ideal Rotational Motion Sensor/LConn1
  C/RConn1 -- Ideal Rotational Motion Sensor/RConn1
  PS-S/LConn1 -- Ideal Rotational Motion Sensor/RConn3

== system ssc_Probes_test_all_16a/dEnergy_2P ==
  PS-S : nesl_utility/PS-Simulink Converter  PhysicalDomain=network_engine_domain  SubClassName=ps_output  LeftPortType=input  RightPortType=output  PseudoPeriodic=off  Frequencies=[]  Unit=kJ/kg  AffineConversion=off
  Pressure & Internal Energy Sensor (2P) : fl_lib/Two-Phase Fluid/Sensors/Pressure & Internal Energy Sensor (2P)
      settings: SourceProductName=Simscape  SourceProductBaseCode=SS  InternalSimscapePortConfiguration="{\"Bottom\":[],\"Left\":[{\"id\":\"A\",\"label\":\"A\",\"type\":\"foundation.two_phase_fluid.two_phase_fluid\"}],\"Right\":[{\"id\":\"B\",\"label\":\"B\",\"type\":\"foundation.two_phase_fluid.two_phase_fluid\"},{\"id\":\"P\",\"label\":\"P\",\"type\":\"output\"},{\"id\":\"U\",\"label\":\"U\",\"type\":\"output\"}],\"Top\":[]}"
  Terminator : Terminator
  A : PMIOPort  Side=Left
  B : PMIOPort  Port=2  Side=Right
  wires:
  PS-S/1 -> [dEnergy_2P]  "dEnergy_2P"
  [dEnergy_2P] -> Terminator/1
  connections:
  Pressure & Internal Energy Sensor (2P)/RConn3 -- PS-S/LConn1
  Pressure & Internal Energy Sensor (2P)/RConn1 -- B/RConn1
  Pressure & Internal Energy Sensor (2P)/LConn1 -- A/RConn1

== system ssc_Probes_test_all_16a/dGasPressure ==
  PS-S : nesl_utility/PS-Simulink Converter  PhysicalDomain=network_engine_domain  SubClassName=ps_output  LeftPortType=input  RightPortType=output  PseudoPeriodic=off  Frequencies=[]  Unit=Pa  AffineConversion=off
  Pneumatic Pressure & Temperature Sensor : Pneumatic_lib/Pneumatic Sensors/Pneumatic Pressure & Temperature Sensor
      settings: InternalSimscapePortConfiguration="{\"Bottom\":[],\"Left\":[{\"id\":\"A\",\"label\":\"A\",\"type\":\"foundation.pneumatic.pneumatic\"}],\"Right\":[{\"id\":\"B\",\"label\":\"B\",\"type\":\"foundation.pneumatic.pneumatic\"},{\"id\":\"P_ps\",\"label\":\"P\",\"type\":\"output\"},{\"id\":\"T_ps\",\"label\":\"T\",\"type\":\"output\"}],\"Top\":[]}"
  Terminator : Terminator
  A : PMIOPort  Side=Left
  B : PMIOPort  Port=2  Side=Right
  wires:
  [dGasPressure] -> Terminator/1
  PS-S/1 -> [dGasPressure]  "dGasPressure"
  connections:
  Pneumatic Pressure & Temperature Sensor/RConn2 -- PS-S/LConn1
  B/RConn1 -- Pneumatic Pressure & Temperature Sensor/RConn1
  A/RConn1 -- Pneumatic Pressure & Temperature Sensor/LConn1

== system ssc_Probes_test_all_16a/dGasTemperature ==
  PS-S : nesl_utility/PS-Simulink Converter  PhysicalDomain=network_engine_domain  SubClassName=ps_output  LeftPortType=input  RightPortType=output  PseudoPeriodic=off  Frequencies=[]  Unit=K  AffineConversion=off
  Pneumatic Pressure & Temperature Sensor : Pneumatic_lib/Pneumatic Sensors/Pneumatic Pressure & Temperature Sensor
      settings: InternalSimscapePortConfiguration="{\"Bottom\":[],\"Left\":[{\"id\":\"A\",\"label\":\"A\",\"type\":\"foundation.pneumatic.pneumatic\"}],\"Right\":[{\"id\":\"B\",\"label\":\"B\",\"type\":\"foundation.pneumatic.pneumatic\"},{\"id\":\"P_ps\",\"label\":\"P\",\"type\":\"output\"},{\"id\":\"T_ps\",\"label\":\"T\",\"type\":\"output\"}],\"Top\":[]}"
  Terminator : Terminator
  A : PMIOPort  Side=Left
  B : PMIOPort  Port=2  Side=Right
  wires:
  [dGasTemperature] -> Terminator/1
  PS-S/1 -> [dGasTemperature]  "dGasTemperature"
  connections:
  A/RConn1 -- Pneumatic Pressure & Temperature Sensor/LConn1
  B/RConn1 -- Pneumatic Pressure & Temperature Sensor/RConn1
  PS-S/LConn1 -- Pneumatic Pressure & Temperature Sensor/RConn3

== system ssc_Probes_test_all_16a/dMMF ==
  MMF Sensor : fl_lib/Magnetic/Magnetic Sensors/MMF Sensor
      settings: SourceProductName=Simscape  SourceProductBaseCode=SS  InternalSimscapePortConfiguration="{\"Bottom\":[],\"Left\":[{\"id\":\"N\",\"label\":\"N\",\"type\":\"foundation.magnetic.magnetic\"}],\"Right\":[{\"id\":\"MMF\",\"label\":\"\",\"type\":\"output\"},{\"id\":\"S\",\"label\":\"S\",\"type\":\"foundation.magnetic.magnetic\"}],\"Top\":[]}"
  PS-S : nesl_utility/PS-Simulink Converter  PhysicalDomain=network_engine_domain  SubClassName=ps_output  LeftPortType=input  RightPortType=output  PseudoPeriodic=off  Frequencies=[]  Unit=A  AffineConversion=off
  Terminator : Terminator
  N : PMIOPort  Side=Left
  S : PMIOPort  Port=2  Side=Right
  wires:
  [dMMF] -> Terminator/1
  PS-S/1 -> [dMMF]  "dMMF"
  connections:
  S/RConn1 -- MMF Sensor/RConn2
  MMF Sensor/RConn1 -- PS-S/LConn1
  N/RConn1 -- MMF Sensor/LConn1

== system ssc_Probes_test_all_16a/dPosition ==
  Ideal Translational Motion Sensor : fl_lib/Mechanical/Mechanical Sensors/Ideal Translational Motion Sensor  offset=0 m
  PS-S : nesl_utility/PS-Simulink Converter  PhysicalDomain=network_engine_domain  SubClassName=ps_output  LeftPortType=input  RightPortType=output  PseudoPeriodic=off  Frequencies=[]  Unit=m  AffineConversion=off
  Terminator : Terminator
  R : PMIOPort  Side=Left
  C : PMIOPort  Port=2  Side=Right
  wires:
  [dPosition] -> Terminator/1
  PS-S/1 -> [dPosition]  "dPosition"
  connections:
  PS-S/LConn1 -- Ideal Translational Motion Sensor/RConn3
  C/RConn1 -- Ideal Translational Motion Sensor/RConn1
  R/RConn1 -- Ideal Translational Motion Sensor/LConn1

== system ssc_Probes_test_all_16a/dPressure ==
  Ideal Hydraulic Pressure Sensor : fl_lib/Hydraulic/Hydraulic Sensors/Hydraulic Pressure Sensor
      settings: SourceProductName=Simscape
  PS-S : nesl_utility/PS-Simulink Converter  PhysicalDomain=network_engine_domain  SubClassName=ps_output  LeftPortType=input  RightPortType=output  PseudoPeriodic=off  Frequencies=[]  Unit=Pa  AffineConversion=off
  Terminator : Terminator
  A : PMIOPort  Side=Left
  B : PMIOPort  Port=2  Side=Right
  wires:
  [dPressure] -> Terminator/1
  PS-S/1 -> [dPressure]  "dPressure"
  connections:
  PS-S/LConn1 -- Ideal Hydraulic Pressure Sensor/RConn2
  B/RConn1 -- Ideal Hydraulic Pressure Sensor/RConn1
  A/RConn1 -- Ideal Hydraulic Pressure Sensor/LConn1

== system ssc_Probes_test_all_16a/dPressure_2P ==
  PS-S : nesl_utility/PS-Simulink Converter  PhysicalDomain=network_engine_domain  SubClassName=ps_output  LeftPortType=input  RightPortType=output  PseudoPeriodic=off  Frequencies=[]  Unit=Pa  AffineConversion=off
  Pressure & Internal Energy Sensor (2P) : fl_lib/Two-Phase Fluid/Sensors/Pressure & Internal Energy Sensor (2P)
      settings: SourceProductName=Simscape  SourceProductBaseCode=SS  InternalSimscapePortConfiguration="{\"Bottom\":[],\"Left\":[{\"id\":\"A\",\"label\":\"A\",\"type\":\"foundation.two_phase_fluid.two_phase_fluid\"}],\"Right\":[{\"id\":\"B\",\"label\":\"B\",\"type\":\"foundation.two_phase_fluid.two_phase_fluid\"},{\"id\":\"P\",\"label\":\"P\",\"type\":\"output\"},{\"id\":\"U\",\"label\":\"U\",\"type\":\"output\"}],\"Top\":[]}"
  Terminator : Terminator
  A : PMIOPort  Side=Left
  B : PMIOPort  Port=2  Side=Right
  wires:
  [dPressure_2P] -> Terminator/1
  PS-S/1 -> [dPressure_2P]  "dPressure_2P"
  connections:
  Pressure & Internal Energy Sensor (2P)/RConn2 -- PS-S/LConn1
  Pressure & Internal Energy Sensor (2P)/LConn1 -- A/RConn1
  Pressure & Internal Energy Sensor (2P)/RConn1 -- B/RConn1

== system ssc_Probes_test_all_16a/dPressure_TL ==
  PS-S : nesl_utility/PS-Simulink Converter  PhysicalDomain=network_engine_domain  SubClassName=ps_output  LeftPortType=input  RightPortType=output  PseudoPeriodic=off  Frequencies=[]  Unit=Pa  AffineConversion=off
  Pressure & Temperature Sensor (TL) : fl_lib/Thermal Liquid/Sensors/Pressure & Temperature Sensor (TL)
      settings: SourceProductName=Simscape  SourceProductBaseCode=SS  InternalSimscapePortConfiguration="{\"Bottom\":[],\"Left\":[{\"id\":\"A\",\"label\":\"A\",\"type\":\"foundation.thermal_liquid.thermal_liquid\"}],\"Right\":[{\"id\":\"B\",\"label\":\"B\",\"type\":\"foundation.thermal_liquid.thermal_liquid\"},{\"id\":\"P\",\"label\":\"P\",\"type\":\"output\"},{\"id\":\"T\",\"label\":\"T\",\"type\":\"output\"}],\"Top\":[]}"
  Terminator : Terminator
  A : PMIOPort  Side=Left
  B : PMIOPort  Port=2  Side=Right
  wires:
  [dPressure_TL] -> Terminator/1
  PS-S/1 -> [dPressure_TL]  "dPressure_TL"
  connections:
  Pressure & Temperature Sensor (TL)/RConn2 -- PS-S/LConn1
  Pressure & Temperature Sensor (TL)/LConn1 -- A/RConn1
  B/RConn1 -- Pressure & Temperature Sensor (TL)/RConn1

== system ssc_Probes_test_all_16a/dTemperature ==
  Ideal Temperature Sensor : fl_lib/Thermal/Thermal Sensors/Temperature Sensor
  PS-S : nesl_utility/PS-Simulink Converter  PhysicalDomain=network_engine_domain  SubClassName=ps_output  LeftPortType=input  RightPortType=output  PseudoPeriodic=off  Frequencies=[]  Unit=K  AffineConversion=off
  Terminator : Terminator
  A : PMIOPort  Side=Left
  B : PMIOPort  Port=2  Side=Right
  wires:
  [dTemperature] -> Terminator/1
  PS-S/1 -> [dTemperature]  "dTemperature"
  connections:
  A/RConn1 -- Ideal Temperature Sensor/LConn1
  B/RConn1 -- Ideal Temperature Sensor/RConn1
  PS-S/LConn1 -- Ideal Temperature Sensor/RConn2

== system ssc_Probes_test_all_16a/dTemperature_TL ==
  PS-S : nesl_utility/PS-Simulink Converter  PhysicalDomain=network_engine_domain  SubClassName=ps_output  LeftPortType=input  RightPortType=output  PseudoPeriodic=off  Frequencies=[]  Unit=K  AffineConversion=off
  Pressure & Temperature Sensor (TL) : fl_lib/Thermal Liquid/Sensors/Pressure & Temperature Sensor (TL)
      settings: SourceProductName=Simscape  SourceProductBaseCode=SS  InternalSimscapePortConfiguration="{\"Bottom\":[],\"Left\":[{\"id\":\"A\",\"label\":\"A\",\"type\":\"foundation.thermal_liquid.thermal_liquid\"}],\"Right\":[{\"id\":\"B\",\"label\":\"B\",\"type\":\"foundation.thermal_liquid.thermal_liquid\"},{\"id\":\"P\",\"label\":\"P\",\"type\":\"output\"},{\"id\":\"T\",\"label\":\"T\",\"type\":\"output\"}],\"Top\":[]}"
  Terminator : Terminator
  A : PMIOPort  Side=Left
  B : PMIOPort  Port=2  Side=Right
  wires:
  PS-S/1 -> [dTemperature_TL]  "dTemperature_TL"
  [dTemperature_TL] -> Terminator/1
  connections:
  PS-S/LConn1 -- Pressure & Temperature Sensor (TL)/RConn3
  B/RConn1 -- Pressure & Temperature Sensor (TL)/RConn1
  Pressure & Temperature Sensor (TL)/LConn1 -- A/RConn1
